simulink model "Project_part2"  (R2024b)
settings: Solver=FixedStepAuto  StartTime=0.0  StopTime=0.1  FixedStep=1e-6  RelTol=1e-3
settings Model: Creator=Talida  LastModifiedBy=Talida
settings SolverCC: EnableFixedStepZeroCrossing=on

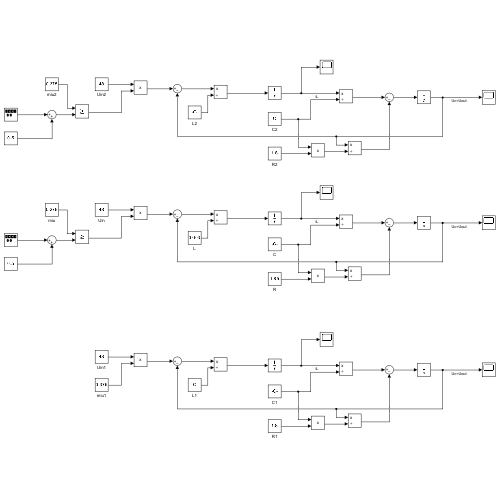
[thumbnail: Simulink's stored preview of the top-level diagram]
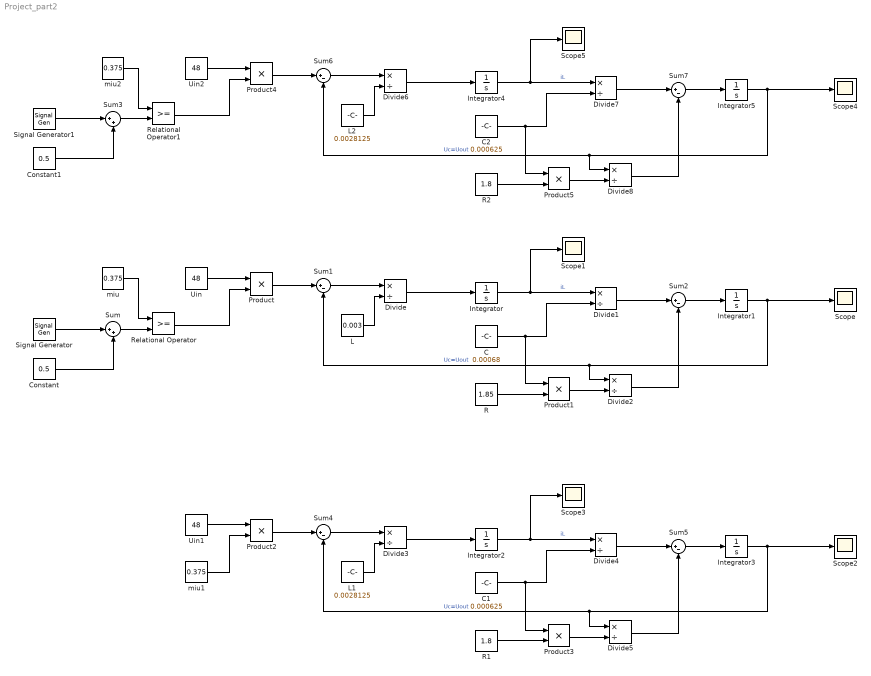
== system Project_part2 ==
  C : Constant  Value=0.00068
  C1 : Constant  Value=0.000625
  C2 : Constant  Value=0.000625
  Constant : Constant  Value=0.5
  Constant1 : Constant  Value=0.5
  Divide{,1..8} (9 alike) : Product  Inputs=*/
  Integrator{,1..5} (6 alike) : Integrator
  L : Constant  Value=0.003
  L1 : Constant  Value=0.0028125
  L2 : Constant  Value=0.0028125
  Product{,1..5} (6 alike) : Product
  R : Constant  Value=1.85
  R1 : Constant  Value=1.8
  R2 : Constant  Value=1.8
  Relational Operator : RelationalOperator  OutDataTypeStr=boolean  RndMeth=Simplest  InputSameDT=off
  Relational Operator1 : RelationalOperator  OutDataTypeStr=boolean  RndMeth=Simplest  InputSameDT=off
  Scope{,1..5} (6 alike) : Scope
  Signal Generator : SignalGenerator  WaveForm=sawtooth  Amplitude=0.5  Frequency=1500
  Signal Generator1 : SignalGenerator  WaveForm=sawtooth  Amplitude=0.5  Frequency=1500
  Sum : Sum  Inputs=|++
  Sum{1..2,4..7} (6 alike) : Sum  Inputs=|+-
  Sum3 : Sum  Inputs=|++
  Uin : Constant  Value=48
  Uin1 : Constant  Value=48
  Uin2 : Constant  Value=48
  miu : Constant  Value=0.375
  miu1 : Constant  Value=0.375
  miu2 : Constant  Value=0.375
  wires:
  Sum3/1 -> Relational Operator1/2
  C1/1 -> Product3/1, Divide4/2
  Divide3/1 -> Integrator2/1
  Signal Generator1/1 -> Sum3/1
  Constant/1 -> Sum/2
  Integrator/1 -> Scope1/1, Divide1/1  "iL"
  Integrator1/1 -> Divide2/1, Sum1/2, Scope/1  "Uc=Uout"
  Sum/1 -> Relational Operator/2
  Signal Generator/1 -> Sum/1
  Divide2/1 -> Sum2/2
  Integrator4/1 -> Scope5/1, Divide7/1  "iL"
  Integrator5/1 -> Divide8/1, Sum6/2, Scope4/1  "Uc=Uout"
  Sum5/1 -> Integrator3/1
  Uin2/1 -> Product4/1
  Product/1 -> Sum1/1
  Divide7/1 -> Sum7/1
  R/1 -> Product1/2
  Uin1/1 -> Product2/1
  Product4/1 -> Sum6/1
  L/1 -> Divide/2
  Sum7/1 -> Integrator5/1
  Product3/1 -> Divide5/2
  Divide6/1 -> Integrator4/1
  Divide4/1 -> Sum5/1
  Divide/1 -> Integrator/1
  Relational Operator1/1 -> Product4/2
  L1/1 -> Divide3/2
  Sum1/1 -> Divide/1
  C2/1 -> Product5/1, Divide7/2
  Divide1/1 -> Sum2/1
  Uin/1 -> Product/1
  Constant1/1 -> Sum3/2
  Integrator3/1 -> Divide5/1, Sum4/2, Scope2/1  "Uc=Uout"
  Integrator2/1 -> Scope3/1, Divide4/1  "iL"
  Divide5/1 -> Sum5/2
  L2/1 -> Divide6/2
  R2/1 -> Product5/2
  Product1/1 -> Divide2/2
  miu/1 -> Relational Operator/1
  Sum6/1 -> Divide6/1
  R1/1 -> Product3/2
  Product2/1 -> Sum4/1
  Sum4/1 -> Divide3/1
  miu1/1 -> Product2/2
  miu2/1 -> Relational Operator1/1
  Sum2/1 -> Integrator1/1
  C/1 -> Product1/1, Divide1/2
  Divide8/1 -> Sum7/2
  Relational Operator/1 -> Product/2
  Product5/1 -> Divide8/2
